simulink model "chap15_1sim"  (Simulink 8.1)
settings: Solver=ode45  StartTime=0.0  StopTime=20  RelTol=1e-3
settings Model: RequirementInfo="{}  %GIDa_76303ea9_e104_4b12_a9d4_ad7d38dcdbab"  Creator=ljk  LastModifiedBy=liujk
settings DataIOCC: SignalLoggingName=sigsOut
settings DebuggingCC: SaveWithParameterizedLinksMsg=none  SignalResolutionControl=TryResolveAllWithWarning  SolverPrmCheckMsg=none  MultiTaskDSMMsg=warning  MultiTaskCondExecSysMsg=none  StrictBusMsg=None
settings HardwareCC: TargetUnknown=on
settings RTWCC: IncludeERTFirstTime=on

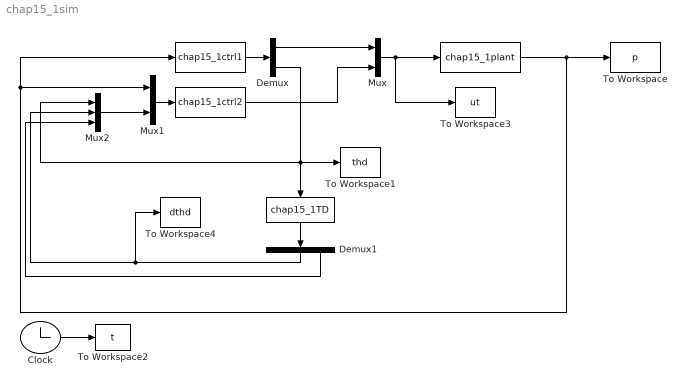
== system chap15_1sim ==
  " " : S-Function  FunctionName=chap15_1TD  EnableBusSupport=off
  "  " : S-Function  FunctionName=chap15_1plant  EnableBusSupport=off
  "    " : S-Function  FunctionName=chap15_1ctrl2  EnableBusSupport=off
  "      " : S-Function  FunctionName=chap15_1ctrl1  EnableBusSupport=off
  Clock : Clock
  Demux : Demux  Outputs=2
  Demux1 : Demux  Outputs=3
  Mux : Mux  Inputs=2
  Mux1 : Mux  Inputs=2
  Mux2 : Mux  Inputs=3
  To Workspace : ToWorkspace  VariableName=p  SampleTime=-1
  To Workspace1 : ToWorkspace  VariableName=thd  SampleTime=-1
  To Workspace2 : ToWorkspace  VariableName=t  SampleTime=-1
  To Workspace3 : ToWorkspace  VariableName=ut  SampleTime=-1
  To Workspace4 : ToWorkspace  VariableName=dthd  SampleTime=-1
  wires:
  Clock/1 -> To Workspace2/1
  "  "/1 -> "      "/1, Mux1/1, To Workspace/1
  Mux/1 -> To Workspace3/1, "  "/1
  "    "/1 -> Mux/2
  "      "/1 -> Demux/1
  Demux/1 -> Mux/1
  Mux1/1 -> "    "/1
  Demux/2 -> To Workspace1/1, " "/1, Mux2/1
  Mux2/1 -> Mux1/2
  " "/1 -> Demux1/1
  Demux1/2 -> To Workspace4/1, Mux2/2
  Demux1/3 -> Mux2/3
